simulink model "laserscan2image"  (R2016a)
settings: Solver=FixedStepAuto  StartTime=0.0  StopTime=inf  RelTol=1e-3
model workspace (MAT data in the model file):
  SL_ROS_VariableLengthArrays_MaxSizes.CommonInfo.ArrayTruncateAction = 'EmitWarning'
  SL_ROS_VariableLengthArrays_MaxSizes.MsgTypeMap = containers.Map
  SL_ROS_VariableLengthArrays_MaxSizes.MsgTypeMap.serialization.keys = {'sensor_msgs/LaserScan'}
  SL_ROS_VariableLengthArrays_MaxSizes.MsgTypeMap.serialization.values{1}(1).PropertyName = 'Ranges'
  SL_ROS_VariableLengthArrays_MaxSizes.MsgTypeMap.serialization.values{1}(1).DataType = 'single'
  SL_ROS_VariableLengthArrays_MaxSizes.MsgTypeMap.serialization.values{1}(1).MaxLength = 180
  SL_ROS_VariableLengthArrays_MaxSizes.MsgTypeMap.serialization.values{1}(2).PropertyName = 'Intensities'
  SL_ROS_VariableLengthArrays_MaxSizes.MsgTypeMap.serialization.values{1}(2).DataType = 'single'
  SL_ROS_VariableLengthArrays_MaxSizes.MsgTypeMap.serialization.values{1}(2).MaxLength = 180
  SL_ROS_VariableLengthArrays_MaxSizes.MsgTypeMap.serialization.uniformity = 0
  SL_ROS_VariableLengthArrays_MaxSizes.MsgTypeMap.serialization.keyType = 'char'
  SL_ROS_VariableLengthArrays_MaxSizes.MsgTypeMap.serialization.valueType = 'any'
libraries: visiongeotforms x1, robotlib x1, visionsinks x1
settings Model: Creator=sprinkle  LastModifiedBy=sprinkle
settings OptimizationCC: OptimizeModelRefInitCode=on  LifeSpan=Inf  MaxStackSize=64
settings HardwareCC: ProdBitPerPointer=32  ProdLargestAtomicFloat=None  ProdIntDivRoundTo=Undefined  ProdEndianess=Unspecified  ProdWordSize=32  ProdHWDeviceType=Generic->Unspecified (assume 32-bit Generic)
settings RTWCC: SystemTargetFile=ert.tlc  HardwareBoard=Robot Operating System (ROS)  TemplateMakefile=ert_default_tmf  GenerateReport=on  Toolchain=Catkin  IncludeHyperlinkInReport=on  LaunchReport=on  TargetLang=C++  GenerateTraceInfo=on  GenerateTraceReport=on  GenerateTraceReportSl=on  GenerateTraceReportSf=on  GenerateTraceReportEml=on
settings CodeAppCC: ForceParamTrailComments=on  IgnoreCustomStorageClasses=off  OperatorAnnotations=on  SimulinkDataObjDesc=on  SFDataObjDesc=on  MATLABFcnDesc=on  InsertBlockDesc=on  MATLABSourceComments=on

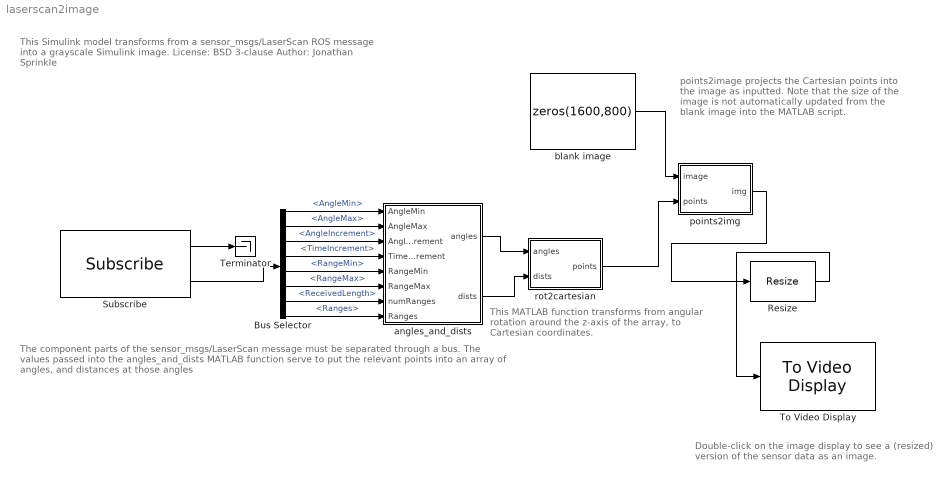
== system laserscan2image ==
  note: The component parts of the sensor_msgs/LaserScan message must be separated
      | through a bus. The values passed into the angles_and_dists MATLAB function serve
      | to put the relevant points into an array of angles, and distances at those angles
  note: This MATLAB function transforms from angular rotation around the z-axis of the array, to Cartesian coordinates.
  note: This Simulink model transforms from a sensor_msgs/LaserScan ROS message into a grayscale Simulink image.
      |
      | License: BSD 3-clause
      | Author: Jonathan Sprinkle
  note: points2image projects the Cartesian points into the image as inputted. Note that the size of the image is not automatically updated from the blank image into the MATLAB script.
  note: Double-click on the image display to see a (resized) version of the sensor data as an image.
  Bus Selector : BusSelector  OutputSignals=AngleMin,AngleMax,AngleIncrement,TimeIncrement,RangeMin,RangeMax,Ranges_SL_Info.ReceivedLength,Ranges
  Resize : visiongeotforms/Resize  specify=Output size as a percentage of input size  rfactor=[25 25]  outCols=25  outRows=25  outRowsCols=[25 35]  interp_method=Bilinear  antialias=on  useROI=off  roiFlag=off  prodOutputMode=Binary point scaling  prodOutputWordLength=32  prodOutputFracLength=10  roundingMode=Nearest  overflowMode=on
  Subscribe : robotlib/Subscribe  SourceLibraryInfo=This block requires Robotics System Toolbox  topicSource=Select from ROS network  topic=/catvehicle/front_laser_points  messageType=sensor_msgs/LaserScan  sampleTime=-1  messageQueueLength=1
  Terminator : Terminator
  To Video Display : visionsinks/To Video Display  windowSizeMode=True size (1:1)  openAtMdlStart=on  fullScreen=off  videoWindowX=0  videoWindowY=-28  saveWindowSize=off  videoWindowWidth=458  videoWindowHeight=1072  inputColorFormat=RGB  inputType=Obsolete  imagePorts=One multidimensional signal  OutputDevice=On-screen video monitor  dataOrg=Column-major  isWindowOpen=off
  angles_and_dists : MATLAB Function  TreatAsAtomicUnit=on
  blank image : Constant  Value=zeros(1600,800)
  points2img : MATLAB Function  TreatAsAtomicUnit=on
  rot2cartesian : MATLAB Function  TreatAsAtomicUnit=on
  wires:
  Subscribe/1 -> Terminator/1
  Subscribe/2 -> Bus Selector/1
  Bus Selector/1 -> angles_and_dists/1(AngleMin)  "<AngleMin>"
  Bus Selector/2 -> angles_and_dists/2(AngleMax)  "<AngleMax>"
  Bus Selector/3 -> angles_and_dists/3(AngleIncrement)  "<AngleIncrement>"
  Bus Selector/4 -> angles_and_dists/4(TimeIncrement)  "<TimeIncrement>"
  Bus Selector/5 -> angles_and_dists/5(RangeMin)  "<RangeMin>"
  Bus Selector/6 -> angles_and_dists/6(RangeMax)  "<RangeMax>"
  Bus Selector/7 -> angles_and_dists/7(numRanges)  "<ReceivedLength>"
  Bus Selector/8 -> angles_and_dists/8(Ranges)  "<Ranges>"
  angles_and_dists/1(angles) -> rot2cartesian/1(angles)
  angles_and_dists/2(dists) -> rot2cartesian/2(dists)
  rot2cartesian/1(points) -> points2img/2(points)
  blank image/1 -> points2img/1(image)
  points2img/1(img) -> Resize/1
  Resize/1 -> To Video Display/1

== matlab function laserscan2image/rot2cartesian ==
  data: angles input; dists input; points output size=[180 2]
function points = fcn(angles,dists)
%#codegen
% x values align with "forward" points
xs = dists.*cos(angles);
% y values align with left (positive) points
ys = dists.*sin(angles);
points = [xs,ys];

== matlab function laserscan2image/angles_and_dists ==
  data: AngleMin input size=1 [-2*pi..2*pi]; angles output size=[180 1]; dists output size=[180 1]; AngleMax input [-2*pi..2*pi]; AngleIncrement input [0..2*pi]; TimeIncrement input; RangeMin input; RangeMax input; numRanges input [1..360]; Ranges input
function [angles,dists] = fcn(AngleMin, AngleMax, AngleIncrement, ...
                TimeIncrement, RangeMin, RangeMax, numRanges, Ranges )
%#codegen
% this function transforms the laser scan into cartesian coordinates, so
% that you can use other tools to group them together, make an image, etc.
if numRanges > 0 
angleMin = double(AngleMin);
angleMax = double(AngleMax);
angleIncrement = double(AngleIncrement);
% assert(angleMax > angleMin);
% assert((angleMax-angleMin)/angleIncrement > 1);

angleMin = -pi/2;
angleMax = pi/2;
angleIncrement = pi/179;
timeIncrement = TimeIncrement;
rangeMin = RangeMin;
rangeMax = RangeMax;
ranges = Ranges;
ranges(ranges>RangeMax) = NaN;
ranges(ranges<RangeMin) = NaN;
%rangesLength = scan.Ranges_SL_Info.ReceivedLength;
%intensities = scan.Intensities;
%coder.varsize('angles',[180 1]);
assert(numRanges < 360);
angles=double(zeros(numRanges,1));
for ii=1:numRanges
    angles(ii) = double(angleMin) + double(ii-1)*(angleIncrement);
end
% angles = [angleMin:angleIncrement:angleMax]';
dists = ranges;
assert(length(dists) == numRanges);
assert(length(dists) == length(angles));
else
    angles=double(0);
    dists=single(0);
end

== matlab function laserscan2image/points2img ==
  data: image input; img output; points input size=[180 2]
function img = fcn(image,points)
%#codegen
img = image;
% we assume we will be getting 180x2 points
len=180;
% the point (0,-20) would, normally, be in the bottom half of the image
% note: (with +x forward, and +y to the left of the car).
% But, the bottom half of the image should be +20 more pixels. So, we will
% instead /subtract/ from 80, all the points. That way, point
pts = points;
% add 80 to all the y points
pts(:,2) = 80 - pts(:,2);
% since we are building an 800x1600 image of the 80m (x) by 160m (y), we
% will multiply the data by 10 and take the floor in order to show
% occupancy near that point
pts = 10*pts;
% iterate over these points, and set up a primitive grid map
for ii=1:len
    ii_x = pts(ii,1); % the x point is in the first column
    ii_y = pts(ii,2); % the y point is in the second comlumn
    if(ii_x > 800)
        disp('ru roh');
    end
    index_x = min(max(10,floor(ii_x)),800-10);
    index_y = min(max(10,floor(ii_y)),1600-10);
    % make a square here, of size 10x10 pixels
    % we must swap the (x,y) to (y,x) for MATLAB images
    img(index_y-5:index_y+5,index_x-5:index_x+5) = ...
        img(index_y-5:index_y+5,index_x-5:index_x+5) | 255;
end
